simulink model "estimator_ekf"  (Simulink 7.0)
settings: Solver=FixedStepDiscrete  StartTime=2  StopTime=2  FixedStep=1e-3  RelTol=1e-3
undefined symbols (not defined in the file): magnitude, P0, Q, R, ROBOT, ts, X0
libraries: simulink x4
settings Model: Creator=raje_ra  LastModifiedBy=raje_ra  ExtModeAutoUpdateStatusClock=off

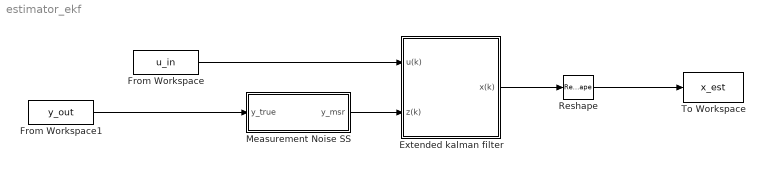
== system estimator_ekf ==
  Extended kalman filter : Subsystem
  From Workspace : FromWorkspace  VariableName=u_in  SampleTime=0
  From Workspace1 : FromWorkspace  VariableName=y_out  SampleTime=0
  Measurement Noise SS : Subsystem
  Reshape : Reshape
  To Workspace : ToWorkspace  VariableName=x_est  SampleTime=-1  SaveFormat=Structure With Time
  wires:
  Extended kalman filter/1(x(k)) -> Reshape/1
  From Workspace1/1 -> Measurement Noise SS/1(y_true)
  From Workspace/1 -> Extended kalman filter/1(u(k))
  Measurement Noise SS/1(y_msr) -> Extended kalman filter/2(z(k))
  Reshape/1 -> To Workspace/1

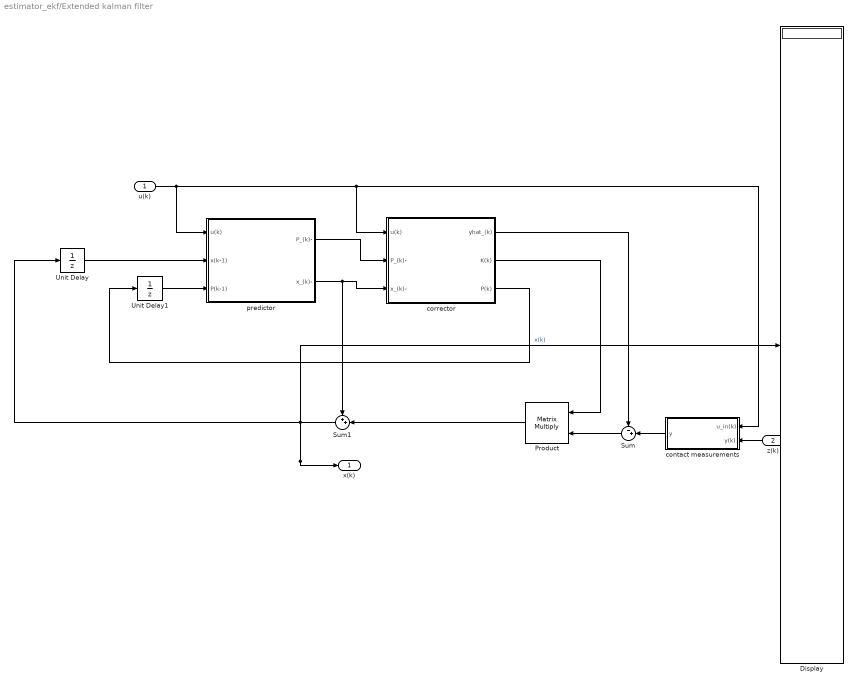
== system estimator_ekf/Extended kalman filter ==
  u(k) : Inport  OutDataType=sfix(16)  OutScaling=2^0
  z(k) : Inport  Orientation=left  Port=2  OutDataType=sfix(16)  OutScaling=2^0
  Display : Display
  Product : Product  Orientation=left  Multiplication=Matrix(*)  OutDataType=sfix(16)  OutScaling=2^0  RndMeth=Zero
  Sum : Sum  Orientation=left  Inputs=-+|  OutDataType=sfix(16)  OutScaling=2^0
  Sum1 : Sum  Orientation=left  Inputs=++|  OutDataType=sfix(16)  OutScaling=2^0
  Unit Delay : UnitDelay  X0=X0  SampleTime=ts
  Unit Delay1 : UnitDelay  X0=P0  SampleTime=ts
  contact measurements : Subsystem  Orientation=left
  corrector : Subsystem
  predictor : Subsystem
  x(k) : Outport  OutDataType=sfix(16)  OutScaling=2^0
  wires:
  u(k)/1 -> predictor/1(u(k)), corrector/1(u(k)), contact measurements/1(u_in(k))
  predictor/2(x_(k)-) -> corrector/3(x_(k)-), Sum1/1
  Unit Delay/1 -> predictor/2(x(k-1))
  corrector/1(yhat_(k)) -> Sum/1
  corrector/2(K(k)) -> Product/1
  Sum/1 -> Product/2
  Unit Delay1/1 -> predictor/3(P(k-1))
  predictor/1(P_(k)-) -> corrector/2(P_(k)-)
  Product/1 -> Sum1/2
  Sum1/1 -> Unit Delay/1, x(k)/1, Display/1  "x(k)"
  corrector/3(P(k)) -> Unit Delay1/1
  contact measurements/1(y) -> Sum/2
  z(k)/1 -> contact measurements/2(y(k))

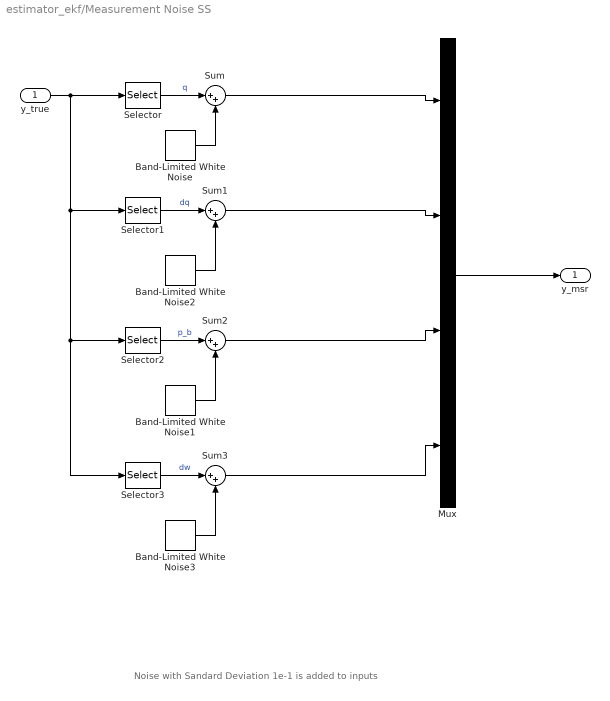
== system estimator_ekf/Measurement Noise SS ==
  note: Noise with Sandard Deviation 1e-1 is added to inputs
  y_true : Inport  OutDataType=sfix(16)  OutScaling=2^0
  Band-Limited White Noise : simulink/Sources/Band-Limited White Noise  SystemSampleTime=-1  Cov=[1e-9]  Ts=ts  seed=[23341]
  Band-Limited White Noise1 : simulink/Sources/Band-Limited White Noise  SystemSampleTime=-1  Cov=[1e-5]  Ts=ts  seed=[23341]
  Band-Limited White Noise2 : simulink/Sources/Band-Limited White Noise  SystemSampleTime=-1  Cov=[1e-7]  Ts=ts  seed=[23341]
  Band-Limited White Noise3 : simulink/Sources/Band-Limited White Noise  SystemSampleTime=-1  Cov=[1e-7]  Ts=ts  seed=[23341]
  Mux : Mux
  Selector : Selector  InputPortWidth=m  IndexOptions=Index vector (dialog)  Indices=[1:25]  OutputSizes=1
  Selector1 : Selector  InputPortWidth=m  IndexOptions=Index vector (dialog)  Indices=[26:50]  OutputSizes=1
  Selector2 : Selector  InputPortWidth=m  IndexOptions=Index vector (dialog)  Indices=[51:53]  OutputSizes=1
  Selector3 : Selector  InputPortWidth=m  IndexOptions=Index vector (dialog)  Indices=[54:56]  OutputSizes=1
  Sum{,1..3} (4 alike) : Sum  Inputs=|++  OutDataType=sfix(16)  OutScaling=2^0
  y_msr : Outport
  wires:
  Band-Limited White Noise/1 -> Sum/2
  y_true/1 -> Selector/1, Selector1/1, Selector2/1, Selector3/1
  Selector/1 -> Sum/1  "q"
  Selector1/1 -> Sum1/1  "dq"
  Band-Limited White Noise2/1 -> Sum1/2
  Band-Limited White Noise1/1 -> Sum2/2
  Selector2/1 -> Sum2/1  "p_b"
  Band-Limited White Noise3/1 -> Sum3/2
  Selector3/1 -> Sum3/1  "dw"
  Sum/1 -> Mux/1
  Sum1/1 -> Mux/2
  Sum2/1 -> Mux/3
  Sum3/1 -> Mux/4
  Mux/1 -> y_msr/1

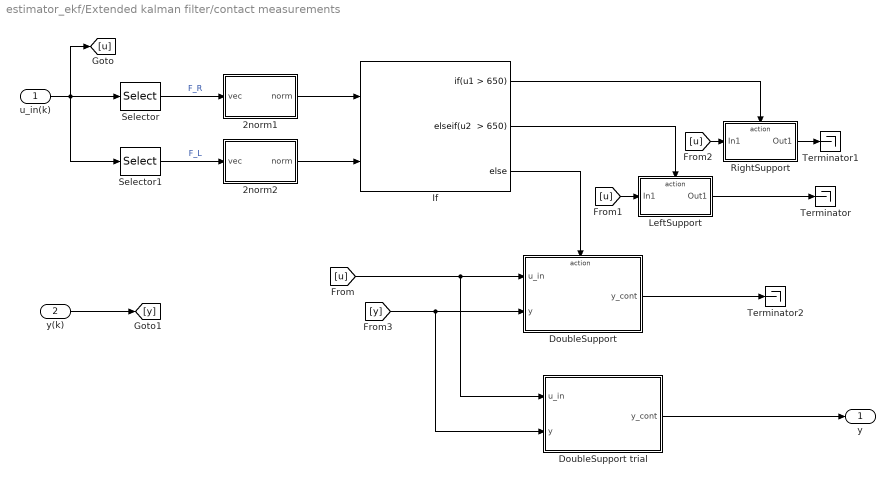
== system estimator_ekf/Extended kalman filter/contact measurements ==
  u_in(k) : Inport
  y(k) : Inport  Port=2
  2norm1 : Subsystem
  2norm2 : Subsystem
  DoubleSupport : Subsystem  TreatAsAtomicUnit=on
  DoubleSupport trial : Subsystem  TreatAsAtomicUnit=on
  If : If  NumInputs=2  IfExpression=u1 > 650  ElseIfExpressions="u2  > 650"
  LeftSupport : Subsystem  TreatAsAtomicUnit=on
  RightSupport : Subsystem  TreatAsAtomicUnit=on
  Selector : Selector  InputPortWidth=37  IndexOptions=Index vector (dialog)  Indices=[1:3]  OutputSizes=1
  Selector1 : Selector  InputPortWidth=37  IndexOptions=Index vector (dialog)  Indices=[4:6]  OutputSizes=1
  Terminator : Terminator
  Terminator1 : Terminator
  Terminator2 : Terminator
  y : Outport
  wires:
  DoubleSupport trial/1(y_cont) -> y/1
  DoubleSupport/1(y_cont) -> Terminator2/1
  LeftSupport/1(Out1) -> Terminator/1
  RightSupport/1(Out1) -> Terminator1/1
  [u] -> DoubleSupport trial/1(u_in), DoubleSupport/1(u_in)
  Selector/1 -> 2norm1/1(vec)  "F_R"
  Selector1/1 -> 2norm2/1(vec)  "F_L"
  2norm1/1(norm) -> If/1
  2norm2/1(norm) -> If/2
  If/1 -> RightSupport/Action
  u_in(k)/1 -> Selector/1, Selector1/1, [u]
  If/3 -> DoubleSupport/Action
  If/2 -> LeftSupport/Action
  [u] -> LeftSupport/1(In1)
  [u] -> RightSupport/1(In1)
  y(k)/1 -> [y]
  [y] -> DoubleSupport trial/2(y), DoubleSupport/2(y)

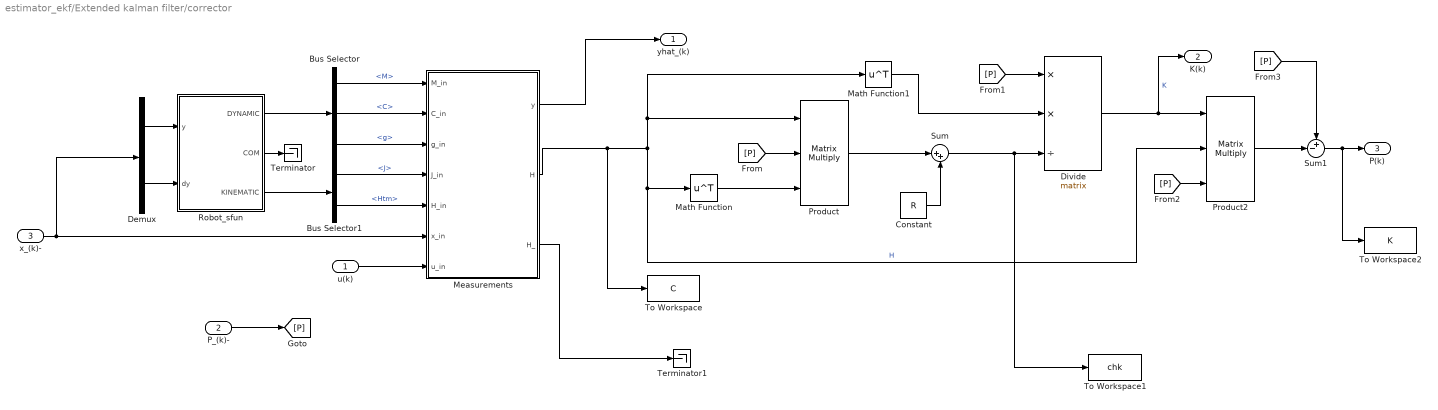
== system estimator_ekf/Extended kalman filter/corrector ==
  u(k) : Inport  OutDataType=sfix(16)  OutScaling=2^0
  P_(k)- : Inport  Port=2  OutDataType=sfix(16)  OutScaling=2^0
  x_(k)- : Inport  Port=3  OutDataType=sfix(16)  OutScaling=2^0
  Bus Selector : BusSelector  OutputSignals=M,C,g
  Bus Selector1 : BusSelector  OutputSignals=J,Htm
  Constant : Constant  Value=R  OutDataType=sfix(16)  OutScaling=2^0
  Demux : Demux  Outputs=2
  Divide : Product  Inputs=**/  Multiplication=Matrix(*)  OutDataType=sfix(16)  OutScaling=2^-10
  Math Function : Math  Operator=transpose  OutDataType=sfix(16)  OutScaling=2^0  SaturateOnIntegerOverflow=on
  Math Function1 : Math  Operator=transpose  OutDataType=sfix(16)  OutScaling=2^0  SaturateOnIntegerOverflow=on
  Measurements : Stateflow chart
  Product : Product  Inputs=3  Multiplication=Matrix(*)  OutDataType=sfix(16)  OutScaling=2^0  RndMeth=Zero
  Product2 : Product  Inputs=3  Multiplication=Matrix(*)  OutDataType=sfix(16)  OutScaling=2^0  RndMeth=Zero
  Robot_sfun : Subsystem
  Sum : Sum  Inputs=|++  OutDataType=sfix(16)  OutScaling=2^0
  Sum1 : Sum  Inputs=+-|  OutDataType=sfix(16)  OutScaling=2^0
  Terminator : Terminator
  Terminator1 : Terminator
  To Workspace : ToWorkspace  VariableName=C  SampleTime=-1  SaveFormat=Array
  To Workspace1 : ToWorkspace  VariableName=chk  SampleTime=-1  SaveFormat=Array
  To Workspace2 : ToWorkspace  VariableName=K  SampleTime=-1  SaveFormat=Array
  yhat_(k) : Outport  OutDataType=sfix(16)  OutScaling=2^0
  K(k) : Outport  Port=2  OutDataType=sfix(16)  OutScaling=2^0
  P(k) : Outport  Port=3  OutDataType=sfix(16)  OutScaling=2^0
  wires:
  Robot_sfun/1(DYNAMIC) -> Bus Selector/1
  Bus Selector/1 -> Measurements/1(M_in)  "<M>"
  Bus Selector/2 -> Measurements/2(C_in)  "<C>"
  Bus Selector/3 -> Measurements/3(g_in)  "<g>"
  Robot_sfun/3(KINEMATIC) -> Bus Selector1/1
  Bus Selector1/1 -> Measurements/4(J_in)  "<J>"
  Bus Selector1/2 -> Measurements/5(H_in)  "<Htm>"
  Demux/1 -> Robot_sfun/1(y)
  Demux/2 -> Robot_sfun/2(dy)
  Robot_sfun/2(COM) -> Terminator/1
  x_(k)-/1 -> Demux/1, Measurements/6(x_in)
  u(k)/1 -> Measurements/7(u_in)
  Math Function/1 -> Product/3
  [P] -> Product/2
  P_(k)-/1 -> [P]
  Product/1 -> Sum/1
  Constant/1 -> Sum/2
  Sum/1 -> Divide/3, To Workspace1/1
  [P] -> Divide/1
  Math Function1/1 -> Divide/2
  Divide/1 -> Product2/1, K(k)/1  "K"
  Measurements/1(y) -> yhat_(k)/1
  [P] -> Product2/3
  [P] -> Sum1/1
  Product2/1 -> Sum1/2
  Sum1/1 -> P(k)/1, To Workspace2/1
  Measurements/3(H_) -> Terminator1/1
  Measurements/2(H) -> Product/1, Math Function1/1, Math Function/1, Product2/2, To Workspace/1  "H"

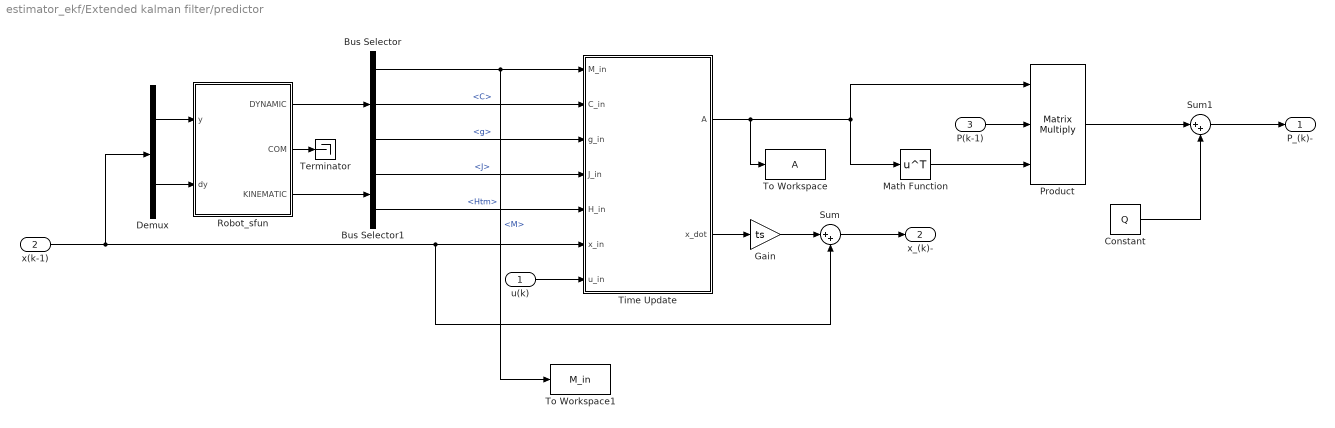
== system estimator_ekf/Extended kalman filter/predictor ==
  u(k) : Inport  OutDataType=sfix(16)  OutScaling=2^0
  x(k-1) : Inport  Port=2  OutDataType=sfix(16)  OutScaling=2^0
  P(k-1) : Inport  Port=3  OutDataType=sfix(16)  OutScaling=2^0
  Bus Selector : BusSelector  OutputSignals=M,C,g
  Bus Selector1 : BusSelector  OutputSignals=J,Htm
  Constant : Constant  Value=Q  OutDataType=sfix(16)  OutScaling=2^0
  Demux : Demux  Outputs=2
  Gain : Gain  Gain=ts  ParameterDataType=sfix(16)  ParameterScaling=2^0  OutDataType=sfix(16)  OutScaling=2^0
  Math Function : Math  Operator=transpose  OutDataType=sfix(16)  OutScaling=2^0  SaturateOnIntegerOverflow=on
  Product : Product  Inputs=3  Multiplication=Matrix(*)  OutDataType=sfix(16)  OutScaling=2^0  RndMeth=Zero
  Robot_sfun : Subsystem
  Sum : Sum  Inputs=|++  OutDataType=sfix(16)  OutScaling=2^0
  Sum1 : Sum  Inputs=|++  OutDataType=sfix(16)  OutScaling=2^0
  Terminator : Terminator
  Time Update : Stateflow chart
  To Workspace : ToWorkspace  VariableName=A  SampleTime=-1  SaveFormat=Array
  To Workspace1 : ToWorkspace  VariableName=M_in  SampleTime=-1  SaveFormat=Array
  P_(k)- : Outport  OutDataType=sfix(16)  OutScaling=2^0
  x_(k)- : Outport  Port=2  OutDataType=sfix(16)  OutScaling=2^0
  wires:
  Robot_sfun/1(DYNAMIC) -> Bus Selector/1
  Bus Selector/1 -> Time Update/1(M_in), To Workspace1/1  "<M>"
  Bus Selector/2 -> Time Update/2(C_in)  "<C>"
  Bus Selector/3 -> Time Update/3(g_in)  "<g>"
  Robot_sfun/3(KINEMATIC) -> Bus Selector1/1
  Bus Selector1/1 -> Time Update/4(J_in)  "<J>"
  Bus Selector1/2 -> Time Update/5(H_in)  "<Htm>"
  x(k-1)/1 -> Demux/1, Time Update/6(x_in), Sum/2
  u(k)/1 -> Time Update/7(u_in)
  Demux/1 -> Robot_sfun/1(y)
  Demux/2 -> Robot_sfun/2(dy)
  Time Update/2(x_dot) -> Gain/1
  Gain/1 -> Sum/1
  Sum/1 -> x_(k)-/1
  Time Update/1(A) -> Math Function/1, Product/1, To Workspace/1
  Math Function/1 -> Product/3
  P(k-1)/1 -> Product/2
  Product/1 -> Sum1/1
  Constant/1 -> Sum1/2
  Sum1/1 -> P_(k)-/1
  Robot_sfun/2(COM) -> Terminator/1

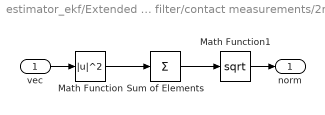
== system estimator_ekf/Extended kalman filter/contact measurements/2norm1 ==
  vec : Inport
  Math Function : Math  Operator=magnitude^2  OutDataType=sfix(16)  OutScaling=2^0  SaturateOnIntegerOverflow=on
  Math Function1 : Math  Operator=sqrt  OutDataType=sfix(16)  OutScaling=2^0  SaturateOnIntegerOverflow=on
  Sum of Elements : Sum  Inputs=+  OutDataType=sfix(16)  OutScaling=2^-10
  norm : Outport
  wires:
  Math Function1/1 -> norm/1
  vec/1 -> Math Function/1
  Sum of Elements/1 -> Math Function1/1
  Math Function/1 -> Sum of Elements/1

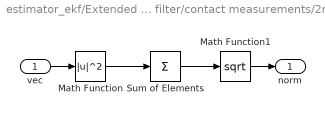
== system estimator_ekf/Extended kalman filter/contact measurements/2norm2 ==
  vec : Inport
  Math Function : Math  Operator=magnitude^2  OutDataType=sfix(16)  OutScaling=2^0  SaturateOnIntegerOverflow=on
  Math Function1 : Math  Operator=sqrt  OutDataType=sfix(16)  OutScaling=2^0  SaturateOnIntegerOverflow=on
  Sum of Elements : Sum  Inputs=+  OutDataType=sfix(16)  OutScaling=2^-10
  norm : Outport
  wires:
  Math Function/1 -> Sum of Elements/1
  Sum of Elements/1 -> Math Function1/1
  vec/1 -> Math Function/1
  Math Function1/1 -> norm/1

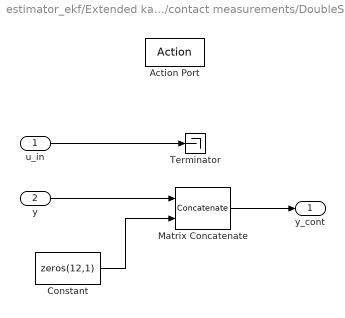
== system estimator_ekf/Extended kalman filter/contact measurements/DoubleSupport ==
  u_in : Inport  OutDataType=sfix(16)  OutScaling=2^0
  y : Inport  Port=2  OutDataType=sfix(16)  OutScaling=2^0
  Action Port : ActionPort  ActionType=else
  Constant : Constant  Value=zeros(12,1)  VectorParams1D=off  OutDataType=sfix(16)  OutScaling=2^0
  Matrix Concatenate : Concatenate  Mode=Multidimensional array
  Terminator : Terminator
  y_cont : Outport  OutDataType=sfix(16)  OutScaling=2^0
  wires:
  u_in/1 -> Terminator/1
  Matrix Concatenate/1 -> y_cont/1
  Constant/1 -> Matrix Concatenate/2
  y/1 -> Matrix Concatenate/1

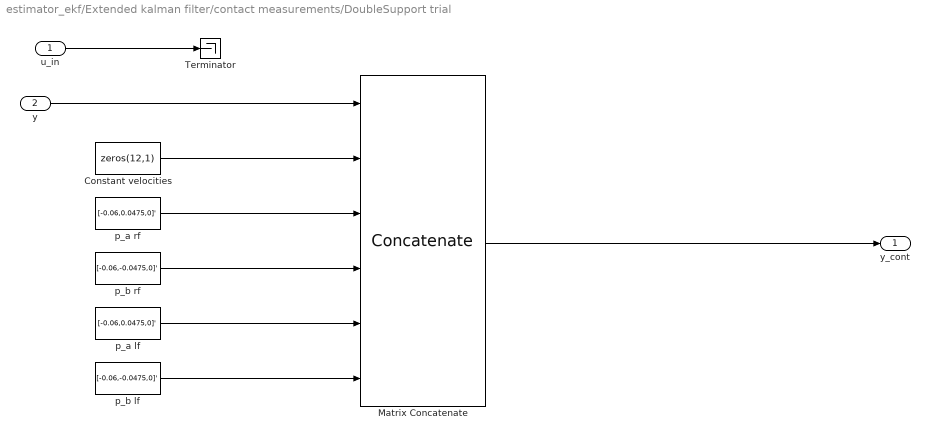
== system estimator_ekf/Extended kalman filter/contact measurements/DoubleSupport trial ==
  u_in : Inport  OutDataType=sfix(16)  OutScaling=2^0
  y : Inport  Port=2  OutDataType=sfix(16)  OutScaling=2^0
  Constant velocities : Constant  Value=zeros(12,1)  VectorParams1D=off  OutDataType=sfix(16)  OutScaling=2^0
  Matrix Concatenate : Concatenate  NumInputs=6  Mode=Multidimensional array
  Terminator : Terminator
  p_a lf : Constant  Value=[-0.06,0.0475,0]'  VectorParams1D=off  OutDataType=sfix(16)  OutScaling=2^0
  p_a rf : Constant  Value=[-0.06,0.0475,0]'  VectorParams1D=off  OutDataType=sfix(16)  OutScaling=2^0
  p_b lf : Constant  Value=[-0.06,-0.0475,0]'  VectorParams1D=off  OutDataType=sfix(16)  OutScaling=2^0
  p_b rf : Constant  Value=[-0.06,-0.0475,0]'  VectorParams1D=off  OutDataType=sfix(16)  OutScaling=2^0
  y_cont : Outport  OutDataType=sfix(16)  OutScaling=2^0
  wires:
  p_a rf/1 -> Matrix Concatenate/3
  y/1 -> Matrix Concatenate/1
  Constant velocities/1 -> Matrix Concatenate/2
  Matrix Concatenate/1 -> y_cont/1
  u_in/1 -> Terminator/1
  p_a lf/1 -> Matrix Concatenate/5
  p_b rf/1 -> Matrix Concatenate/4
  p_b lf/1 -> Matrix Concatenate/6

== system estimator_ekf/Extended kalman filter/contact measurements/LeftSupport ==
  In1 : Inport  OutDataType=sfix(16)  OutScaling=2^0
  Action Port : ActionPort  ActionType=elseif
  Out1 : Outport  OutDataType=sfix(16)  OutScaling=2^0
  wires:
  In1/1 -> Out1/1

== system estimator_ekf/Extended kalman filter/contact measurements/RightSupport ==
  In1 : Inport  OutDataType=sfix(16)  OutScaling=2^0
  Action Port : ActionPort  ActionType=then
  Out1 : Outport  OutDataType=sfix(16)  OutScaling=2^0
  wires:
  In1/1 -> Out1/1

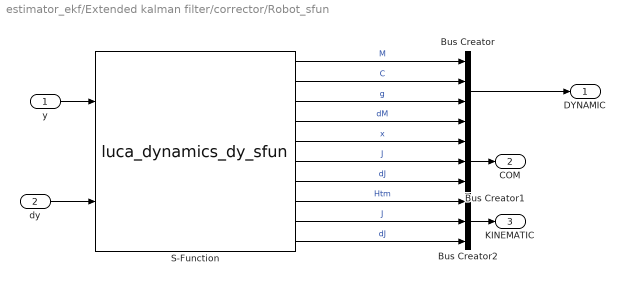
== system estimator_ekf/Extended kalman filter/corrector/Robot_sfun ==
  y : Inport
  dy : Inport  Port=2
  Bus Creator : BusCreator
  Bus Creator1 : BusCreator  Inputs=3
  Bus Creator2 : BusCreator  Inputs=3
  S-Function : S-Function  FunctionName=luca_dynamics_dy_sfun  Parameters=(size(ROBOT.csi,1)/6-1), size(ROBOT.csi,2), ROBOT.parent, ROBOT.tcp, ROBOT.g0, ROBOT.csi, ROBOT.com, ROBOT.Mass
  DYNAMIC : Outport
  COM : Outport  Port=2
  KINEMATIC : Outport  Port=3
  wires:
  y/1 -> S-Function/1
  dy/1 -> S-Function/2
  S-Function/1 -> Bus Creator/1  "M"
  S-Function/2 -> Bus Creator/2  "C"
  S-Function/3 -> Bus Creator/3  "g"
  S-Function/4 -> Bus Creator/4  "dM"
  S-Function/5 -> Bus Creator1/1  "x"
  S-Function/6 -> Bus Creator1/2  "J"
  S-Function/7 -> Bus Creator1/3  "dJ"
  S-Function/8 -> Bus Creator2/1  "Htm"
  S-Function/9 -> Bus Creator2/2  "J"
  S-Function/10 -> Bus Creator2/3  "dJ"
  Bus Creator/1 -> DYNAMIC/1
  Bus Creator1/1 -> COM/1
  Bus Creator2/1 -> KINEMATIC/1

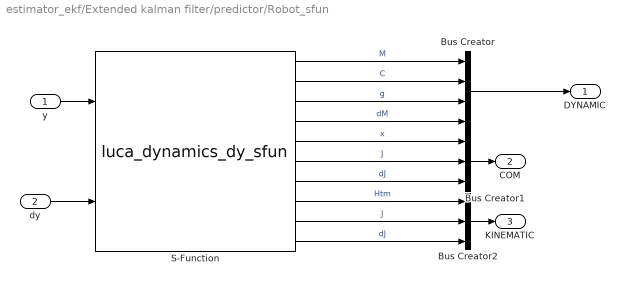
== system estimator_ekf/Extended kalman filter/predictor/Robot_sfun ==
  y : Inport
  dy : Inport  Port=2
  Bus Creator : BusCreator
  Bus Creator1 : BusCreator  Inputs=3
  Bus Creator2 : BusCreator  Inputs=3
  S-Function : S-Function  FunctionName=luca_dynamics_dy_sfun  Parameters=(size(ROBOT.csi,1)/6-1), size(ROBOT.csi,2), ROBOT.parent, ROBOT.tcp, ROBOT.g0, ROBOT.csi, ROBOT.com, ROBOT.Mass
  DYNAMIC : Outport
  COM : Outport  Port=2
  KINEMATIC : Outport  Port=3
  wires:
  Bus Creator2/1 -> KINEMATIC/1
  Bus Creator1/1 -> COM/1
  Bus Creator/1 -> DYNAMIC/1
  S-Function/10 -> Bus Creator2/3  "dJ"
  S-Function/9 -> Bus Creator2/2  "J"
  S-Function/8 -> Bus Creator2/1  "Htm"
  S-Function/7 -> Bus Creator1/3  "dJ"
  S-Function/6 -> Bus Creator1/2  "J"
  S-Function/5 -> Bus Creator1/1  "x"
  S-Function/4 -> Bus Creator/4  "dM"
  S-Function/3 -> Bus Creator/3  "g"
  S-Function/2 -> Bus Creator/2  "C"
  S-Function/1 -> Bus Creator/1  "M"
  dy/1 -> S-Function/2
  y/1 -> S-Function/1

== matlab function Extended kalman filter/predictor/Time Update ==
  data: A output inherited; M_in input inherited; x_dot output inherited; C_in input inherited; g_in input inherited; J_in input inherited; H_in input inherited; x_in input inherited; u_in input inherited
function [A,x_dot]= fcn(M_in,C_in,g_in,J_in,H_in,x_in,u_in)
% This block supports the Embedded MATLAB subset.
% See the help menu for details. 
%Ja = zeros(62,62);
%Extract the matrices from input
debug = 0;
M = M_in(1:31,:);
C = C_in(1:31,:);
g = g_in(1:31);
Jr = J_in(1:6,:);
Jl = J_in(7:12,:);
J_fb = J_in(25:30,:);
H_sb = H_in(17:19,:);
x = x_in;
p = x_in(1:31);
v = x_in(32:62);
Fr = u_in(1:6);
Fl = u_in(7:12);
tau = [zeros(6,1); u_in(13:37)];

% Transformation matrix for the rotational velocity of floating base
T_ori = [1 0 sin(p(5)); 0 cos(p(4)) -cos(p(5))*sin(p(4)); 0 sin(p(4)) cos(p(5))*cos(p(4))];
T = [eye(3),zeros(3);zeros(3),T_ori];

% Transformation from body to spacial frame:

Adj_sb = Adjoint(H_sb);

% Transformation for the velocites of floating base
vbase = T \ (Adj_sb*v(1:6));

vel = [vbase; v(7:31)];

% Computation of accelerations
B = (-C*v - g + tau + Jr'*Fr + Jl'*Fl);
acc = M \ B;

x_dot = [vel;acc];

% used to print output to the the command window in debug mode.
if debug
    H_sb
    T_ori
    Adj_sb
    M
    rank(M)
    C
    g
    Jr
    Jl
end
    

% Computation of Jacobian for velocities of Floating base
dp = Jvbase(p(1:6),v(1:6),Adj_sb,J_fb,T);                    %%%%%%%%%%%%%%%%         
dq = [zeros(25,37),eye(25)];                               %%%%%%%%%%%%%%%%

% Compute the Jacobian of acceleration terms(forward dynamics):
dacc = zeros(31,62);
for i = 1:62
    dM = M_in(i*31+(1:31),:);
    dC = C_in(i*31+(1:31),:);
    dg = g_in(i*31+(1:31));
    dJr = J_in(i*30+(1:6),:);
    dJl = J_in(i*30+(7:12),:);
    if i <= 31
        df = -M^(-1)*dM*M^(-1)*B + M^(-1)*(-dC*v - dg + dJr'*Fr + dJl'*Fl);
    else
        df = -M^(-1)*dM*M^(-1)*B + M^(-1)*(-dC*v - C(:,i-31));
    end
    dacc(:,i) = df;
end
A = [dp;dq;dacc];

== matlab function Extended kalman filter/corrector/Measurements ==
  data: M_in input inherited; y output inherited; C_in input inherited; g_in input inherited; J_in input inherited; H_in input inherited; x_in input inherited; u_in input inherited; H output inherited; H_ output inherited
function [y,H,H_]= fcn(M_in,C_in,g_in,J_in,H_in,x_in,u_in)
% This block supports the Embedded MATLAB subset.
% See the help menu for details. 

debug = 1;
%Extract the matrices from input
M = M_in(1:31,:);
C = C_in(1:31,:);
g = g_in(1:31);
Jr = J_in(1:6,:);
Jl = J_in(7:12,:);
Jb = J_in(25:30,:);
H_sb = H_in(17:19,:);
H_sr = H_in(1:3,:);
H_sl = H_in(5:7,:);
R_sb = H_in(17:19,1:3);
x = x_in;
p = x_in(1:31);
v = x_in(32:62);
omega = v(4:6);
Fr = u_in(1:6);
Fl = u_in(7:12);
tau = [zeros(6,1); u_in(13:37)];


% Transformation matrix to obtain rotational velocity of floating base from
% angular velocity.
T = [1 0 sin(p(5)); 0 cos(p(4)) -sin(p(4))*cos(p(5)); 0 sin(p(4)) cos(p(4))*cos(p(5))];
%T = [eye(3),zeros(3);zeros(3),T_ori];

% Transformation from body to spacial frame:
Adj_sb = Adjoint(H_sb);
inv_Adj = InvAdjoint(H_sb);

% Transformation for the velocites of floating base
%vbase = T \ (Adj_sb*v(1:6));
%vbase_msr = inv_Adj*vbase; 
msr_gyro = R_sb'*T^(-1)*R_sb*omega;

% Computation of accelerations
B = (-C*v - g + tau + Jr'*Fr + Jl'*Fl);
acc = M \ B;

msr_j = [p(7:31);v(7:31)];

% Accleration measurement with the compensation of gravity
msr_pacc = acc(1:3) + R_sb'*[0 0 9.81]';

% Velocity measurements for foot contact
v_rf = Jr*v; 
v_lf = Jl*v;
msr_vcont = [v_rf;v_lf];

% Position of the contact points
pa_s_rf = [-0.06 -0.06545 -1.164279056 1]';
pb_s_rf = [-0.06 -0.1605 -1.164279056 1]';
pa_s_lf = [-0.06 0.1605 -1.164279056 1]';
pb_s_lf = [-0.06 0.06545 -1.164279056 1]';
%H_ap = [eye(3) [-0.06,0.0475,0]'; 0 0 0 1];
%pa_rf = mulH(InvH(H_ap),InvH(H_rf))*[p(1:3);1];
pa_b_rf = InvH(H_sr)*pa_s_rf;
pb_b_rf = InvH(H_sr)*pb_s_rf;
pa_b_lf = InvH(H_sl)*pa_s_lf;
pb_b_lf = InvH(H_sl)*pb_s_lf;
msr_pcont = [pa_b_rf(1:3);pb_b_rf(1:3);pa_b_lf(1:3);pb_b_lf(1:3)];

%measurement equation 
y = [msr_j;msr_pacc;msr_gyro;msr_pcont;msr_vcont];

% Compute the Jacobian of acceleration terms(forward dynamics):
dacc = zeros(3,62);
for i = 1:62
    dM = M_in(i*31+(1:31),:);
    dC = C_in(i*31+(1:31),:);
    dg = g_in(i*31+(1:31));
    dJr = J_in(i*30+(1:6),:);
    dJl = J_in(i*30+(7:12),:);
    dR_sb = H_in(i*20+(17:19),1:3);
    if i <= 31
        df = -M^(-1)*dM*acc+ M^(-1)*(-dC*v - dg + dJr'*Fr + dJl'*Fl);     % acc= M\B;
    else
        df = -M^(-1)*dM*acc + M^(-1)*(-dC*v - C(:,i-31));
    end
    dacc(1:3,i) = df(1:3)+dR_sb'*[0 0 9.81]';
end

% Computing Jacobinan for gyro
% dvbase = Jvbase(p(1:6),v(1:6),Adj_sb,Jb,T);
 dgyro = zeros(3,62);
% adj_J = zeros(6);
% temp = zeros(6,1);
% for i = 1:31    
%     adj_J = Adj_vel(Jb,i);
%     temp = -adj_J*inv_Adj*vbase;
%     dgyro(:,i)  = temp(4:6);
% end
% aux = inv_Adj*dvbase;
% dgyro = dgyro + aux(4:6,:);
dTx = [0 0 0; 0 -sin(p(4)) -cos(p(4))*cos(p(5)); 0 cos(p(4)) -sin(p(4))*cos(p(5))];
dTy = [0 0 cos(p(5)); 0 0 sin(p(4))*sin(p(5)); 0 0 -cos(p(4))*sin(p(5))];
dT = [dTx;dTy;zeros(3)];
temp2 = eye(3);
for i = 1:37
    dR_sb = H_in(i*20+(17:19),1:3);
    if (i <= 3) || (i >= 7 && i <= 31)
        dgyro(:,i) = dR_sb'*T^(-1)*R_sb*omega + R_sb'*T^(-1)*dR_sb*omega;
    elseif i >= 4 && i <= 6
        dgyro(:,i) = dR_sb'*T^(-1)*R_sb*omega - R_sb'*T^(-1)*dT((i-4)*3+(1:3),:)*T^(-1)*R_sb*omega ...
        + R_sb'*T^(-1)*dR_sb*omega;
    elseif i >= 35
        temp2 = R_sb'*T^(-1)*R_sb;
        dgyro(:,i) = temp2(:,i-34);
    end 
end

% Computing Jacobians for foot contact velocities
dvcont = zeros(12,62);
dpcont = zeros(12,62);
temp1 = zeros(16,1);
for i = 1:37
    dJr = J_in(i*30+(1:6),:);
    dJl = J_in(i*30+(7:12),:);
    dHsr = H_in(i*20+(1:4),:);
    dHsl = H_in(i*20+(5:8),:);
    if i <= 31
        dvcont(:,i) = [dJr;dJl]*v;
        temp1 = [-InvH(H_sr)*dHsr*InvH(H_sr)*pa_s_rf; -InvH(H_sr)*dHsr*InvH(H_sr)*pb_s_rf; ...
                 -InvH(H_sl)*dHsl*InvH(H_sl)*pa_s_lf; -InvH(H_sl)*dHsl*InvH(H_sl)*pb_s_lf];
        dpcont(:,i) = [temp1(1:3);temp1(5:7);temp1(9:11);temp1(13:15)];
    elseif i>31 && i <= 37
        dvcont(:,i) = [dJr(:,i-31);dJl(:,i-31)];
    end
end


djp = [zeros(25,6),eye(25),zeros(25,31)];
djv = [zeros(25,37),eye(25)];

% Measurement matrix
H = [djp;djv;dacc;dgyro;dpcont;dvcont];

%%%% Test observability
Jacbase = [eye(6),zeros(6,56)];
%H_ = [Jacbase;dqp;dqv;dacc;dgyro];
H_ = [djp;djv;dacc;dgyro;dpcont];
